simulink model "Chap7_3sim"  (R2019a)
settings: Solver=VariableStepAuto  StartTime=0.0  StopTime=30  MaxStep=.01  RelTol=1e-3
settings Model: Creator=zkibria  LastModifiedBy=zkibria

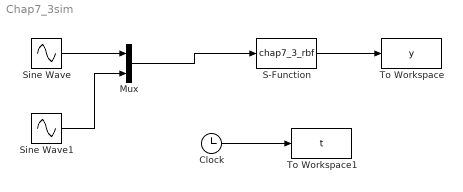
== system Chap7_3sim ==
  Clock : Clock
  Mux : Mux  Inputs=2
  S-Function : S-Function  FunctionName=chap7_3_rbf  SFunctionDeploymentMode=off  EnableBusSupport=off
  Sine Wave : Sin  SampleTime=0
  Sine Wave1 : Sin  SampleTime=0
  To Workspace : ToWorkspace  VariableName=y  SaveFormat=Timeseries  SampleTime=-1
  To Workspace1 : ToWorkspace  VariableName=t  SaveFormat=Timeseries  SampleTime=-1
  wires:
  S-Function/1 -> To Workspace/1
  Clock/1 -> To Workspace1/1
  Sine Wave/1 -> Mux/1
  Sine Wave1/1 -> Mux/2
  Mux/1 -> S-Function/1
